simulink model "Li_ion_cell_p2d_with_control_R2021b"  (R2021b)
settings: Solver=FixedStepDiscrete  StartTime=0.0  StopTime=t_end  FixedStep=dt  RelTol=1e-3
values from neighbouring files (symbols this model uses):
  Const = 0.065777522687874415    [LIB_p2d_dictionary.sldd]
  dt = 0.5    [LIB_p2d_dictionary.sldd]    (also in P2D_run.m = data.t_s(II,1) - data.t_s(II-1,1))
undefined symbols (not defined in the file or in its folder): t_eoc, V_max, xn_init, xp_init
libraries: simulink x4
settings Model: Creator=simba  LastModifiedBy=simba
settings DebuggingCC: ParameterPrecisionLossMsg=none  UnconnectedInputMsg=none  UnconnectedOutputMsg=none  UnconnectedLineMsg=none
settings ModelReferenceCC: EnableRefExpFcnMdlSchedulingChecks=off
settings RTWCC: GPUComputeCapability=5.0  DLArmComputeVersion=20.02.1
settings ConfigComp: CovBoundaryAbsTol=1.0e-5

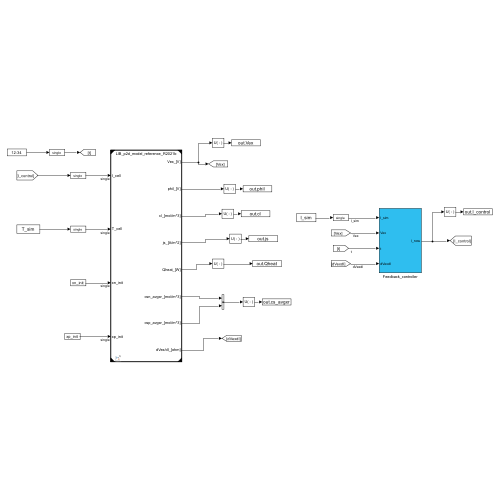
[thumbnail: Simulink's stored preview of the top-level diagram]
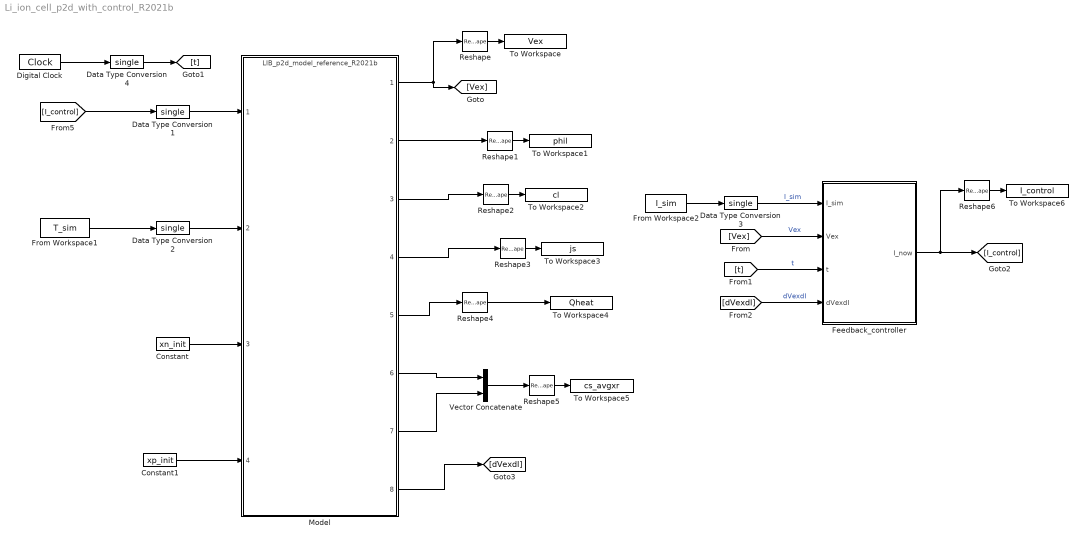
== system Li_ion_cell_p2d_with_control_R2021b ==
  Constant : Constant  Value=xn_init  OutDataTypeStr=single
  Constant1 : Constant  Value=xp_init  OutDataTypeStr=single
  Data Type Conversion{1..4} (4 alike) : DataTypeConversion  OutDataTypeStr=single
  Digital Clock : DigitalClock  SampleTime=dt
  Feedback_controller : Subsystem
  From Workspace1 : FromWorkspace  VariableName=T_sim  SampleTime=dt
  From Workspace2 : FromWorkspace  VariableName=I_sim  SampleTime=dt
  Model : ModelReference  ModelNameDialog=LIB_p2d_model_reference_R2021b.slx  SimulationMode=Accelerator  ModelReferenceVersion=1.0
  Reshape{,1..6} (7 alike) : Reshape
  To Workspace : ToWorkspace  VariableName=Vex  SaveFormat=Timeseries  SampleTime=-1
  To Workspace1 : ToWorkspace  VariableName=phil  SaveFormat=Timeseries  SampleTime=-1
  To Workspace2 : ToWorkspace  VariableName=cl  SaveFormat=Timeseries  SampleTime=-1
  To Workspace3 : ToWorkspace  VariableName=js  SaveFormat=Timeseries  SampleTime=-1
  To Workspace4 : ToWorkspace  VariableName=Qheat  SaveFormat=Timeseries  SampleTime=-1
  To Workspace5 : ToWorkspace  VariableName=cs_avgxr  SaveFormat=Timeseries  SampleTime=-1
  To Workspace6 : ToWorkspace  VariableName=I_control  SaveFormat=Timeseries  SampleTime=-1
  Vector Concatenate : Concatenate
  wires:
  Digital Clock/1 -> Data Type Conversion4/1
  Data Type Conversion1/1 -> Model/1
  From Workspace1/1 -> Data Type Conversion2/1
  Data Type Conversion2/1 -> Model/2
  Constant/1 -> Model/3
  Constant1/1 -> Model/4
  Model/1 -> Reshape/1, [Vex]
  From Workspace2/1 -> Data Type Conversion3/1
  Data Type Conversion4/1 -> [t]
  Model/8 -> [dVexdI]
  [I_control] -> Data Type Conversion1/1
  Data Type Conversion3/1 -> Feedback_controller/1(I_sim)  "I_sim"
  [Vex] -> Feedback_controller/2(Vex)  "Vex"
  [t] -> Feedback_controller/3(t)  "t"
  [dVexdI] -> Feedback_controller/4(dVexdI)  "dVexdI"
  Feedback_controller/1(I_now) -> Reshape6/1, [I_control]
  Reshape/1 -> To Workspace/1
  Model/2 -> Reshape1/1
  Reshape1/1 -> To Workspace1/1
  Model/3 -> Reshape2/1
  Reshape2/1 -> To Workspace2/1
  Model/4 -> Reshape3/1
  Reshape3/1 -> To Workspace3/1
  Model/5 -> Reshape4/1
  Reshape4/1 -> To Workspace4/1
  Vector Concatenate/1 -> Reshape5/1
  Model/6 -> Vector Concatenate/1
  Model/7 -> Vector Concatenate/2
  Reshape5/1 -> To Workspace5/1
  Reshape6/1 -> To Workspace6/1

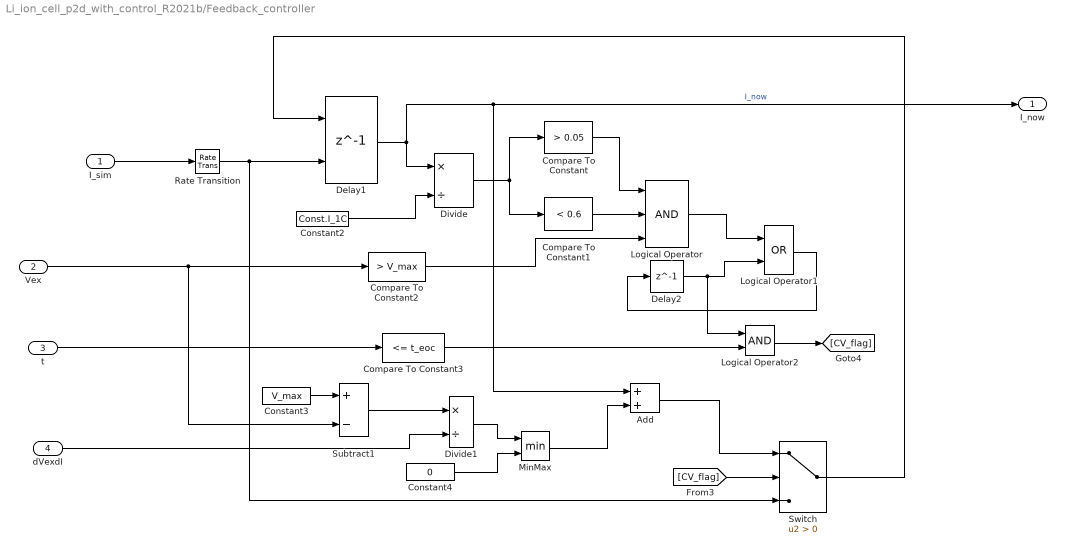
== system Li_ion_cell_p2d_with_control_R2021b/Feedback_controller ==
  I_sim : Inport
  Vex : Inport  Port=2
  t : Inport  Port=3
  dVexdI : Inport  Port=4
  Add : Sum
  Compare To Constant : simulink/Logic and Bit Operations/Compare To Constant  relop=>  const=0.05  OutDataTypeStr=boolean
  Compare To Constant1 : simulink/Logic and Bit Operations/Compare To Constant  relop=<  const=0.6  OutDataTypeStr=boolean
  Compare To Constant2 : simulink/Logic and Bit Operations/Compare To Constant  relop=>  const=V_max  OutDataTypeStr=boolean
  Compare To Constant3 : simulink/Logic and Bit Operations/Compare To Constant  relop=<=  const=t_eoc  OutDataTypeStr=boolean
  Constant2 : Constant  Value=Const.I_1C  OutDataTypeStr=single
  Constant3 : Constant  Value=V_max  OutDataTypeStr=single
  Constant4 : Constant  Value=0  OutDataTypeStr=single
  Delay1 : Delay  DelayLength=1  InitialConditionSource=Input port  InitialCondition=0
      settings: InputPortMap=u0,p4
  Delay2 : Delay  DelayLength=1  InitialCondition=0
  Divide : Product  Inputs=*/
  Divide1 : Product  Inputs=*/
  Logical Operator : Logic  Inputs=3  AllPortsSameDT=off  OutDataTypeStr=boolean
  Logical Operator1 : Logic  Operator=OR  AllPortsSameDT=off  OutDataTypeStr=boolean
  Logical Operator2 : Logic  AllPortsSameDT=off  OutDataTypeStr=boolean
  MinMax : MinMax  Inputs=2
  Rate Transition : RateTransition  OutPortSampleTime=dt
  Subtract1 : Sum  Inputs=+-
  Switch : Switch  Criteria=u2 > Threshold
  I_now : Outport
  wires:
  Delay2/1 -> Logical Operator2/1, Logical Operator1/2
  Delay1/1 -> Add/1, I_now/1, Divide/1  "I_now"
  Divide1/1 -> MinMax/1
  Divide/1 -> Compare To Constant1/1, Compare To Constant/1
  Constant4/1 -> MinMax/2
  Logical Operator2/1 -> [CV_flag]
  Rate Transition/1 -> Delay1/2, Switch/3
  Logical Operator/1 -> Logical Operator1/1
  Compare To Constant1/1 -> Logical Operator/2
  Subtract1/1 -> Divide1/1
  Vex/1 -> Subtract1/2, Compare To Constant2/1
  t/1 -> Compare To Constant3/1
  MinMax/1 -> Add/2
  Constant3/1 -> Subtract1/1
  Compare To Constant/1 -> Logical Operator/1
  Compare To Constant2/1 -> Logical Operator/3
  Logical Operator1/1 -> Delay2/1
  dVexdI/1 -> Divide1/2
  Compare To Constant3/1 -> Logical Operator2/2
  Constant2/1 -> Divide/2
  Add/1 -> Switch/1
  [CV_flag] -> Switch/2
  Switch/1 -> Delay1/1
  I_sim/1 -> Rate Transition/1
